simulink model "sysSim"  (R2017a)
settings: Solver=VariableStepAuto  StartTime=0.0  StopTime=Tsim  RelTol=1e-3
values from neighbouring files (symbols this model uses):
  A = [0.6 1 0 2 0; 0 0.5 0.3 1.5 3; 0 0 0.8 0 3; 0 0 0 0.7 1 ... (first row only)    [fullOrderObs.m]    (also in redOrderObs.m; sysSim.m)
  B = [0 0; 0 0; 1 0; 0 0; 0 1]    [fullOrderObs.m]    (also in redOrderObs.m; sysSim.m)
  C = [1 0 0 0 0 ; 0 1 0 0 0 ]    [fullOrderObs.m]    (also in redOrderObs.m; sysSim.m)
  D = [0 0; 0 0]    [fullOrderObs.m]    (also in redOrderObs.m; sysSim.m)
  step1 = 1    [fullOrderObs.m]    (also in redOrderObs.m; sysSim.m)
  step2 = 2    [fullOrderObs.m]    (also in redOrderObs.m; sysSim.m)
  Ts = 1    [fullOrderObs.m]    (also in redOrderObs.m; sysSim.m)
  x0 = [0 0 0 0 0]    [fullOrderObs.m]    (also in redOrderObs.m; sysSim.m)
settings Model: Creator=clafuno  LastModifiedBy=clafuno

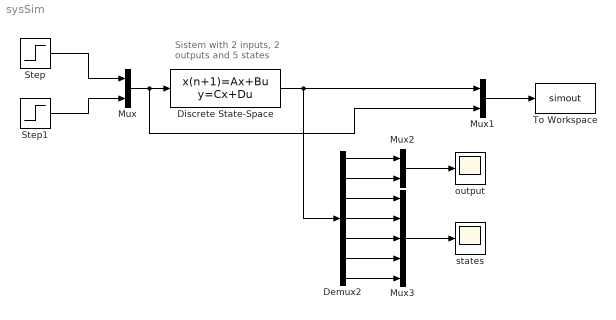
== system sysSim ==
  note: Sistem with 2 inputs, 2 outputs and 5 states
  Demux2 : Demux  Outputs=7
  Discrete State-Space : DiscreteStateSpace  A=A  B=B  C=[C;eye(5)]  D=[D;zeros(5,2)]  X0=x0  SampleTime=Ts
  Mux : Mux  Inputs=2
  Mux1 : Mux  Inputs=2
  Mux2 : Mux  Inputs=2
  Mux3 : Mux  Inputs=5
  Step : Step  After=step1  SampleTime=Ts
  Step1 : Step  After=step2  SampleTime=Ts
  To Workspace : ToWorkspace  VariableName=simout  SampleTime=Ts
  output : Scope
  states : Scope
  wires:
  Mux/1 -> Mux1/2, Discrete State-Space/1
  Step/1 -> Mux/1
  Step1/1 -> Mux/2
  Mux1/1 -> To Workspace/1
  Discrete State-Space/1 -> Mux1/1, Demux2/1
  Demux2/1 -> Mux2/1
  Demux2/2 -> Mux2/2
  Demux2/5 -> Mux3/3
  Demux2/4 -> Mux3/2
  Demux2/3 -> Mux3/1
  Demux2/6 -> Mux3/4
  Demux2/7 -> Mux3/5
  Mux2/1 -> output/1
  Mux3/1 -> states/1
